simulink model "Burner_TestBed1_org"  (Simulink 10.0)
settings: Solver=FixedStepDiscrete  StartTime=0.0  StopTime=1  FixedStep=1  RelTol=1e-3  EnableMultiTasking=on
undefined symbols (not defined in the file): MWS
libraries: Lib_Turbo_Burner_TMATS x1
settings Model: Creator=jwchapm2  LastModifiedBy=bhisma
settings DataIOCC: LimitDataPoints=on
settings OptimizationCC: ExpressionDepthLimit=2147483647
settings DebuggingCC: SolverPrmCheckMsg=warning  StateNameClashWarn=warning
settings GRTTargetCC: GeneratePreprocessorConditionals=Disable all  CombineOutputUpdateFcns=on  GRTInterface=off
settings ConfigComp: CovExternalEMLEnable=off

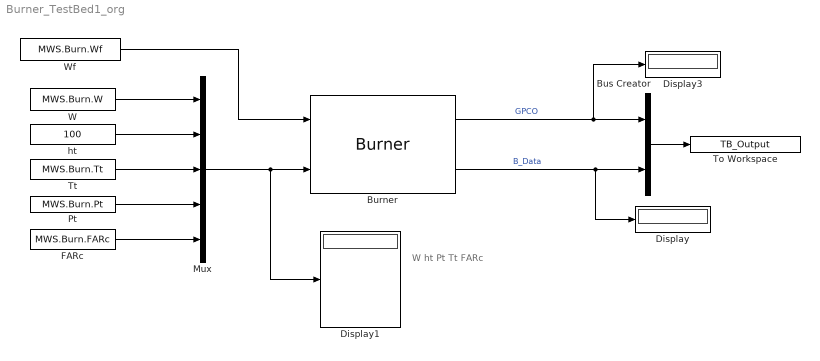
== system Burner_TestBed1_org ==
  note: W
      | ht
      | Pt
      | Tt
      | FARc
  Burner : Lib_Turbo_Burner_TMATS/Burner  LHV_M=MWS.Burn.LHV  dPnormBurner_M=MWS.Burn.dP
  Bus Creator : BusCreator  Inputs=2
  Display : Display
  Display1 : Display
  Display3 : Display
  FARc : Constant  Value=MWS.Burn.FARc
  Mux : Mux  Inputs=5
  Pt : Constant  Value=MWS.Burn.Pt
  To Workspace : ToWorkspace  VariableName=TB_Output  SampleTime=-1
  Tt : Constant  Value=MWS.Burn.Tt
  W : Constant  Value=MWS.Burn.W
  Wf : Constant  Value=MWS.Burn.Wf
  ht : Constant  Value=100
  wires:
  W/1 -> Mux/1
  FARc/1 -> Mux/5
  Tt/1 -> Mux/3
  Pt/1 -> Mux/4
  Mux/1 -> Display1/1, Burner/2
  Burner/1 -> Display3/1, Bus Creator/1  "GPCO"
  Burner/2 -> Display/1, Bus Creator/2  "B_Data"
  Bus Creator/1 -> To Workspace/1
  ht/1 -> Mux/2
  Wf/1 -> Burner/1
